simulink model "Modelado_pendulo"  (R2023a)
settings: Solver=VariableStepAuto  StartTime=0.0  StopTime=10  MaxStep=0.0001  RelTol=1e-3
values from neighbouring files (symbols this model uses):
  g = 9.81    [Pendulo.m]
  l1 = 0.3    [Pendulo.m]
  l2 = 0.25    [Pendulo.m]
  m1 = 0.2    [Pendulo.m]
  m2 = 0.1    [Pendulo.m]
settings Model: Creator=mluser  LastModifiedBy=alcal
settings OptimizationCC: ReuseModelBlockBuffer=off

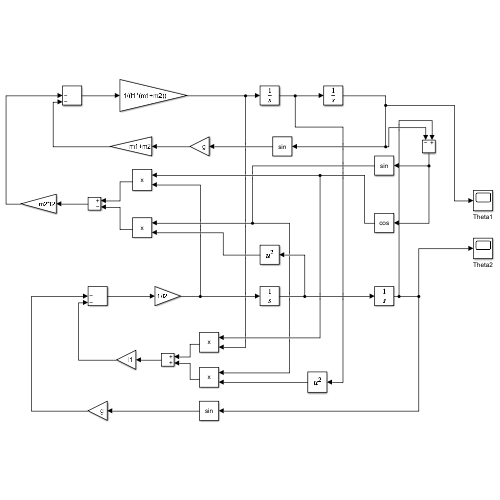
[thumbnail: Simulink's stored preview of the top-level diagram]
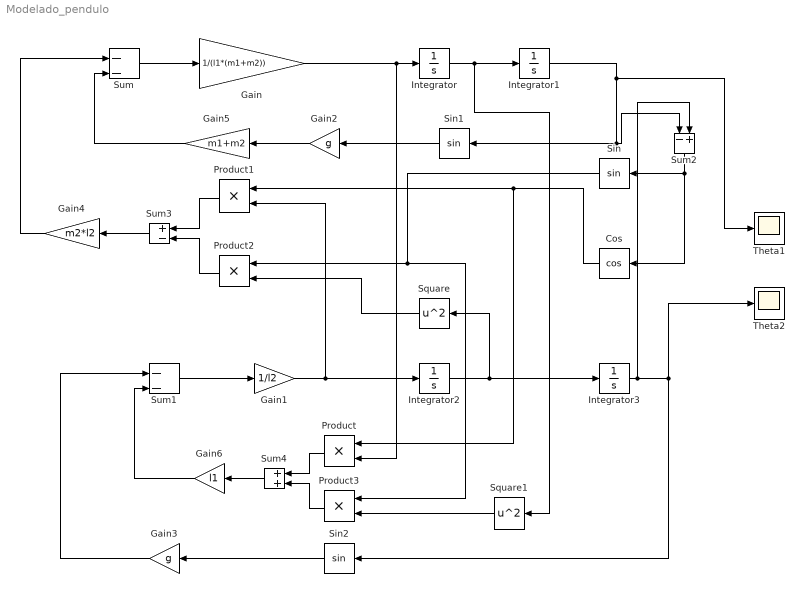
== system Modelado_pendulo ==
  Cos : Trigonometry  Operator=cos
  Gain : Gain  Gain=1/(l1*(m1+m2))
  Gain1 : Gain  Gain=1/l2
  Gain2 : Gain  Gain=g
  Gain3 : Gain  Gain=g
  Gain4 : Gain  Gain=m2*l2
  Gain5 : Gain  Gain=m1+m2
  Gain6 : Gain  Gain=l1
  Integrator : Integrator
  Integrator1 : Integrator
  Integrator2 : Integrator
  Integrator3 : Integrator  InitialCondition=(35*pi)/180
  Product{,1..3} (4 alike) : Product
  Sin : Trigonometry
  Sin1 : Trigonometry
  Sin2 : Trigonometry
  Square : Math  Operator=square
  Square1 : Math  Operator=square
  Sum : Sum  Inputs=|--
  Sum1 : Sum  Inputs=|--
  Sum2 : Sum  Inputs=-+
  Sum3 : Sum  Inputs=+-
  Sum4 : Sum
  Theta1 : Scope
  Theta2 : Scope
  wires:
  Integrator/1 -> Square1/1, Integrator1/1
  Sum/1 -> Gain/1
  Integrator1/1 -> Theta1/1, Sin1/1, Sum2/1
  Gain/1 -> Product/2, Integrator/1
  Integrator2/1 -> Integrator3/1, Square/1
  Sum1/1 -> Gain1/1
  Gain1/1 -> Product1/2, Integrator2/1
  Integrator3/1 -> Sin2/1, Theta2/1, Sum2/2
  Sum2/1 -> Cos/1, Sin/1
  Cos/1 -> Product/1, Product1/1
  Sin/1 -> Product3/1, Product2/1
  Square/1 -> Product2/2
  Product1/1 -> Sum3/1
  Product2/1 -> Sum3/2
  Sum3/1 -> Gain4/1
  Sin1/1 -> Gain2/1
  Gain2/1 -> Gain5/1
  Gain4/1 -> Sum/1
  Product/1 -> Sum4/1
  Product3/1 -> Sum4/2
  Sin2/1 -> Gain3/1
  Gain3/1 -> Sum1/1
  Square1/1 -> Product3/2
  Sum4/1 -> Gain6/1
  Gain6/1 -> Sum1/2
  Gain5/1 -> Sum/2
